simulink model "arlht_lu"  (R2020a)
settings: Solver=FixedStepDiscrete  StartTime=0.0  StopTime=inf  RelTol=1e-3
InitFcn:
  | % Clear workspace
  | clc; clear; close all;
  | 
  | fs = 250e6;
  | 
  | % Set parameters
  | height = 768;
  | width = 1024;
  | sobelThreshold = 30;
  | dTheta = 180/104;
  | theta = (0:dTheta:180-dTheta);
  | 
  | % Derive variables
  | maxRho = ceil(sqrt((height/2)^2+(width/2)^2));
  | nRho = maxRho*2;
  | nTheta = length(theta);
  | 
  | % Read in image and resize
  | I = imread('chess.jpg');
  | Ir = imresize(I, [height, width]);
  | 
  | % Get greyscale
  | Y = rgb2gray(Ir);
  | 
  | % Get Sobel and Gradient
  | [edge, dir, mag] = SobelEdge(Y, 100);
  | dirNew = floor(dir/dTheta)*dTheta;
  | simDirNew = dirNew*2^16;
  | simDirNew(edge==0) = 255*2^16;
  | 
  | % Create input array
  | inarray = uint32(simDirNew);
StopFcn:
  | [hps, Aopt, rbm] = ARLHT(edge, dirNew, dTheta, 1, 0, 4);
  | plot3DHPS(hps);
  | 
  | simHps = reshape(out.simout, [nRho, nTheta]);
  | plot3DHPS(simHps);
values from neighbouring files (symbols this model uses):
  dir = rad2deg(atan(Gy./Gx))    [SobelEdge.m]
libraries: simulink x53, hdlsllib x37, library x3, dspsrcs4 x1
(part 2 of 2)

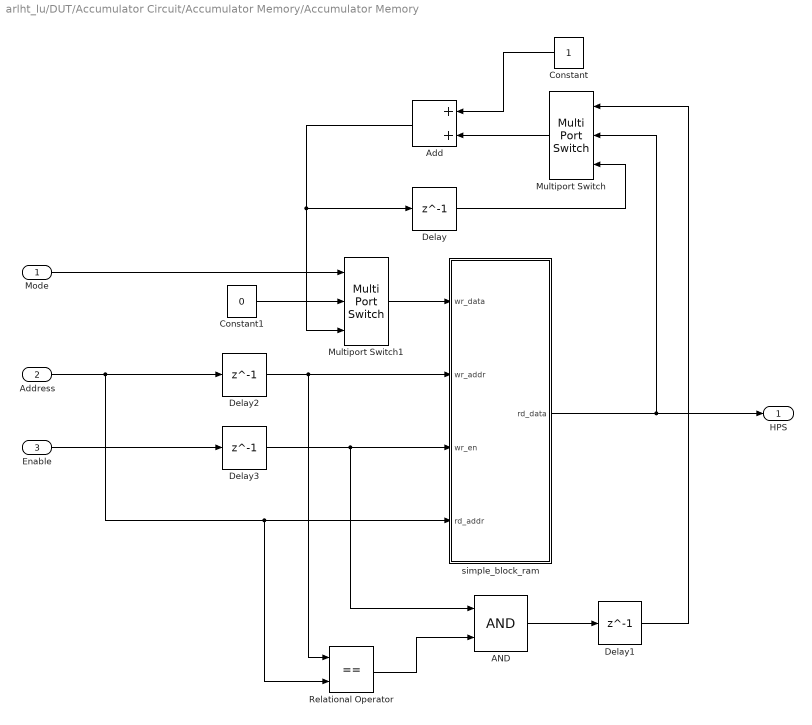
== system arlht_lu/DUT/Accumulator Circuit/Accumulator Memory/Accumulator Memory ==
  Mode : Inport
  Address : Inport  Port=2
  Enable : Inport  Port=3
  AND : Logic  IconShape=distinctive  AllPortsSameDT=off  OutDataTypeStr=boolean
  Add : Sum  OutDataTypeStr=fixdt(0,rhoBits,0)
  Constant : Constant  OutDataTypeStr=fixdt(0,1,0)  SampleTime=-1
  Constant1 : Constant  Value=0  OutDataTypeStr=fixdt(0,rhoBits,0)  SampleTime=-1
  Delay{,1..3} (4 alike) : Delay  DelayLength=1
  Multiport Switch : MultiPortSwitch  DataPortOrder=Zero-based contiguous  Inputs=2  zeroidx=on
  Multiport Switch1 : MultiPortSwitch  DataPortOrder=Zero-based contiguous  Inputs=2  zeroidx=on
  Relational Operator : RelationalOperator  Operator===  OutDataTypeStr=boolean  RndMeth=Simplest
  simple_block_ram : Subsystem  VariantControl=other_bits  mask{b=rhoBits, d=nRho*nTheta/kTheta, b_hidden=36, d_hidden=33280}
      mask prompts: b "Data width:"; d "Depth:"
      mask init: same as arlht_lu/DUT/RBM Circuit/Accumulator Memory/simple_block_ram
  HPS : Outport
  wires:
  Mode/1 -> Multiport Switch1/1
  Multiport Switch1/1 -> simple_block_ram/1(wr_data)
  Address/1 -> Relational Operator/2, simple_block_ram/4(rd_addr), Delay2/1
  simple_block_ram/1(rd_data) -> HPS/1, Multiport Switch/2
  AND/1 -> Delay1/1
  Delay/1 -> Multiport Switch/3
  Multiport Switch/1 -> Add/2
  Delay2/1 -> Relational Operator/1, simple_block_ram/2(wr_addr)
  Constant/1 -> Add/1
  Constant1/1 -> Multiport Switch1/2
  Add/1 -> Multiport Switch1/3, Delay/1
  Delay3/1 -> AND/1, simple_block_ram/3(wr_en)
  Relational Operator/1 -> AND/2
  Enable/1 -> Delay3/1
  Delay1/1 -> Multiport Switch/1

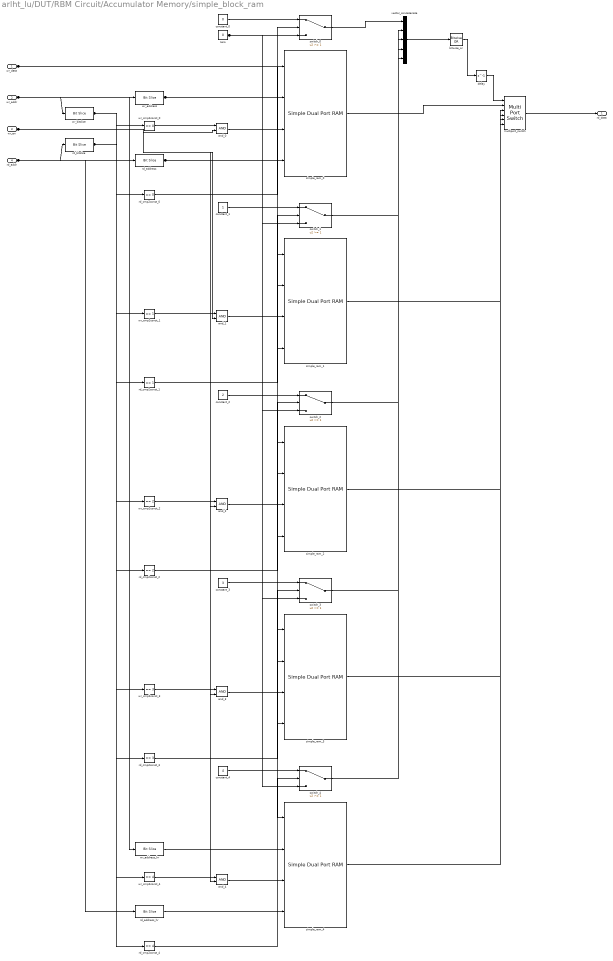
== system arlht_lu/DUT/RBM Circuit/Accumulator Memory/simple_block_ram ==
  wr_data : Inport
  wr_addr : Inport  Port=2
  wr_en : Inport  Port=3
  rd_addr : Inport  Port=4
  and_{0..4} (5 alike) : Logic  AllPortsSameDT=off  OutDataTypeStr=boolean
  bitwise_or : simulink/Logic and Bit Operations/Bitwise Operator  logicop=OR  UseBitMask=off  BitMask=bin2dec('11011001')  BitMaskRealWorld=Stored Integer
  constant_0 : Constant  Value=0  OutDataTypeStr=fixdt(0, 5, 0)  SampleTime=-1
  constant_1 : Constant  OutDataTypeStr=fixdt(0, 5, 0)  SampleTime=-1
  constant_2 : Constant  Value=2  OutDataTypeStr=fixdt(0, 5, 0)  SampleTime=-1
  constant_3 : Constant  Value=3  OutDataTypeStr=fixdt(0, 5, 0)  SampleTime=-1
  constant_4 : Constant  Value=4  OutDataTypeStr=fixdt(0, 5, 0)  SampleTime=-1
  delay : Delay  DelayLength=1
  multiport_switch : MultiPortSwitch  DataPortOrder=Zero-based contiguous  Inputs=5  zeroidx=on
  rd_address : hdlsllib/Logic and Bit Operations/Bit Slice  lidx=14  ridx=0
      settings: SourceProductBaseCode=SL
  rd_address_hr : hdlsllib/Logic and Bit Operations/Bit Slice  lidx=13  ridx=0
      settings: SourceProductBaseCode=SL
  rd_bitslice : hdlsllib/Logic and Bit Operations/Bit Slice  lidx=17  ridx=15
      settings: SourceProductBaseCode=SL
  rd_cmp2const_0 : simulink/Logic and Bit Operations/Compare To Constant  relop===  const=0  OutDataTypeStr=boolean
  rd_cmp2const_1 : simulink/Logic and Bit Operations/Compare To Constant  relop===  const=1  OutDataTypeStr=boolean
  rd_cmp2const_2 : simulink/Logic and Bit Operations/Compare To Constant  relop===  const=2  OutDataTypeStr=boolean
  rd_cmp2const_3 : simulink/Logic and Bit Operations/Compare To Constant  relop===  const=3  OutDataTypeStr=boolean
  rd_cmp2const_4 : simulink/Logic and Bit Operations/Compare To Constant  relop===  const=4  OutDataTypeStr=boolean
  simple_ram_{0..3} (4 alike) : hdlsllib/HDL RAMs/Simple Dual Port RAM  ram_size=15
      settings: SourceProductBaseCode=SL
  simple_ram_4 : hdlsllib/HDL RAMs/Simple Dual Port RAM  ram_size=14
      settings: SourceProductBaseCode=SL
  switch_{0..4} (5 alike) : Switch  Threshold=1
  vector_concatenate : Concatenate  NumInputs=5
  wr_address : hdlsllib/Logic and Bit Operations/Bit Slice  lidx=14  ridx=0
      settings: SourceProductBaseCode=SL
  wr_address_hr : hdlsllib/Logic and Bit Operations/Bit Slice  lidx=13  ridx=0
      settings: SourceProductBaseCode=SL
  wr_bitslice : hdlsllib/Logic and Bit Operations/Bit Slice  lidx=17  ridx=15
      settings: SourceProductBaseCode=SL
  wr_cmp2const_0 : simulink/Logic and Bit Operations/Compare To Constant  relop===  const=0  OutDataTypeStr=boolean
  wr_cmp2const_1 : simulink/Logic and Bit Operations/Compare To Constant  relop===  const=1  OutDataTypeStr=boolean
  wr_cmp2const_2 : simulink/Logic and Bit Operations/Compare To Constant  relop===  const=2  OutDataTypeStr=boolean
  wr_cmp2const_3 : simulink/Logic and Bit Operations/Compare To Constant  relop===  const=3  OutDataTypeStr=boolean
  wr_cmp2const_4 : simulink/Logic and Bit Operations/Compare To Constant  relop===  const=4  OutDataTypeStr=boolean
  zero : Constant  Value=0  OutDataTypeStr=fixdt(0, 5, 0)  SampleTime=-1
  rd_data : Outport
  wires:
  wr_data/1 -> simple_ram_0/1, simple_ram_1/1, simple_ram_2/1, simple_ram_3/1, simple_ram_4/1
  wr_address/1 -> simple_ram_0/2, simple_ram_1/2, simple_ram_2/2, simple_ram_3/2
  rd_address/1 -> simple_ram_0/4, simple_ram_1/4, simple_ram_2/4, simple_ram_3/4
  constant_0/1 -> switch_0/1
  zero/1 -> switch_0/3, switch_1/3, switch_2/3, switch_3/3, switch_4/3
  switch_0/1 -> vector_concatenate/1
  simple_ram_0/1 -> multiport_switch/2
  wr_bitslice/1 -> wr_cmp2const_0/1, wr_cmp2const_1/1, wr_cmp2const_2/1, wr_cmp2const_3/1, wr_cmp2const_4/1
  rd_bitslice/1 -> rd_cmp2const_0/1, rd_cmp2const_1/1, rd_cmp2const_2/1, rd_cmp2const_3/1, rd_cmp2const_4/1
  wr_en/1 -> and_0/2, and_1/2, and_2/2, and_3/2, and_4/2
  and_0/1 -> simple_ram_0/3
  wr_cmp2const_0/1 -> and_0/1
  rd_cmp2const_0/1 -> switch_0/2
  constant_1/1 -> switch_1/1
  switch_1/1 -> vector_concatenate/2
  simple_ram_1/1 -> multiport_switch/3
  and_1/1 -> simple_ram_1/3
  wr_cmp2const_1/1 -> and_1/1
  rd_cmp2const_1/1 -> switch_1/2
  constant_2/1 -> switch_2/1
  switch_2/1 -> vector_concatenate/3
  simple_ram_2/1 -> multiport_switch/4
  and_2/1 -> simple_ram_2/3
  wr_cmp2const_2/1 -> and_2/1
  rd_cmp2const_2/1 -> switch_2/2
  constant_3/1 -> switch_3/1
  switch_3/1 -> vector_concatenate/4
  simple_ram_3/1 -> multiport_switch/5
  and_3/1 -> simple_ram_3/3
  wr_cmp2const_3/1 -> and_3/1
  rd_cmp2const_3/1 -> switch_3/2
  constant_4/1 -> switch_4/1
  switch_4/1 -> vector_concatenate/5
  simple_ram_4/1 -> multiport_switch/6
  and_4/1 -> simple_ram_4/3
  wr_cmp2const_4/1 -> and_4/1
  rd_cmp2const_4/1 -> switch_4/2
  rd_addr/1 -> rd_bitslice/1, rd_address/1, rd_address_hr/1
  wr_addr/1 -> wr_bitslice/1, wr_address/1, wr_address_hr/1
  vector_concatenate/1 -> bitwise_or/1
  bitwise_or/1 -> delay/1
  delay/1 -> multiport_switch/1
  multiport_switch/1 -> rd_data/1
  wr_address_hr/1 -> simple_ram_4/2
  rd_address_hr/1 -> simple_ram_4/4

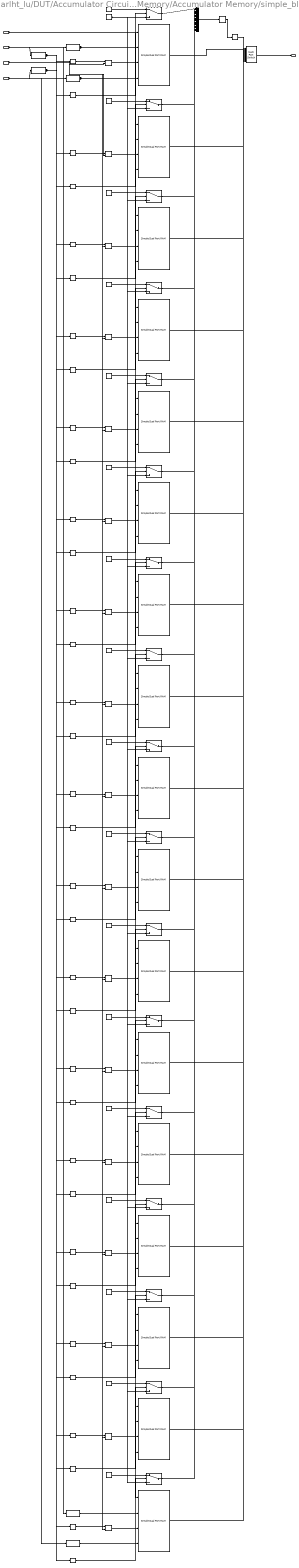
== system arlht_lu/DUT/Accumulator Circuit/Accumulator Memory/Accumulator Memory/simple_block_ram ==
  wr_data : Inport
  wr_addr : Inport  Port=2
  wr_en : Inport  Port=3
  rd_addr : Inport  Port=4
  and_{0..16} (17 alike) : Logic  AllPortsSameDT=off  OutDataTypeStr=boolean
  bitwise_or : simulink/Logic and Bit Operations/Bitwise Operator  logicop=OR  UseBitMask=off  BitMask=bin2dec('11011001')  BitMaskRealWorld=Stored Integer
  constant_0 : Constant  Value=0  OutDataTypeStr=fixdt(0, 17, 0)  SampleTime=-1
  constant_1 : Constant  OutDataTypeStr=fixdt(0, 17, 0)  SampleTime=-1
  constant_10 : Constant  Value=10  OutDataTypeStr=fixdt(0, 17, 0)  SampleTime=-1
  constant_11 : Constant  Value=11  OutDataTypeStr=fixdt(0, 17, 0)  SampleTime=-1
  constant_12 : Constant  Value=12  OutDataTypeStr=fixdt(0, 17, 0)  SampleTime=-1
  constant_13 : Constant  Value=13  OutDataTypeStr=fixdt(0, 17, 0)  SampleTime=-1
  constant_14 : Constant  Value=14  OutDataTypeStr=fixdt(0, 17, 0)  SampleTime=-1
  constant_15 : Constant  Value=15  OutDataTypeStr=fixdt(0, 17, 0)  SampleTime=-1
  constant_16 : Constant  Value=16  OutDataTypeStr=fixdt(0, 17, 0)  SampleTime=-1
  constant_2 : Constant  Value=2  OutDataTypeStr=fixdt(0, 17, 0)  SampleTime=-1
  constant_3 : Constant  Value=3  OutDataTypeStr=fixdt(0, 17, 0)  SampleTime=-1
  constant_4 : Constant  Value=4  OutDataTypeStr=fixdt(0, 17, 0)  SampleTime=-1
  constant_5 : Constant  Value=5  OutDataTypeStr=fixdt(0, 17, 0)  SampleTime=-1
  constant_6 : Constant  Value=6  OutDataTypeStr=fixdt(0, 17, 0)  SampleTime=-1
  constant_7 : Constant  Value=7  OutDataTypeStr=fixdt(0, 17, 0)  SampleTime=-1
  constant_8 : Constant  Value=8  OutDataTypeStr=fixdt(0, 17, 0)  SampleTime=-1
  constant_9 : Constant  Value=9  OutDataTypeStr=fixdt(0, 17, 0)  SampleTime=-1
  delay : Delay  DelayLength=1
  multiport_switch : MultiPortSwitch  DataPortOrder=Zero-based contiguous  Inputs=17  zeroidx=on
  rd_address : hdlsllib/Logic and Bit Operations/Bit Slice  lidx=10  ridx=0
      settings: SourceProductBaseCode=SL
  rd_address_hr : hdlsllib/Logic and Bit Operations/Bit Slice  lidx=9  ridx=0
      settings: SourceProductBaseCode=SL
  rd_bitslice : hdlsllib/Logic and Bit Operations/Bit Slice  lidx=15  ridx=11
      settings: SourceProductBaseCode=SL
  rd_cmp2const_0 : simulink/Logic and Bit Operations/Compare To Constant  relop===  const=0  OutDataTypeStr=boolean
  rd_cmp2const_1 : simulink/Logic and Bit Operations/Compare To Constant  relop===  const=1  OutDataTypeStr=boolean
  rd_cmp2const_10 : simulink/Logic and Bit Operations/Compare To Constant  relop===  const=10  OutDataTypeStr=boolean
  rd_cmp2const_11 : simulink/Logic and Bit Operations/Compare To Constant  relop===  const=11  OutDataTypeStr=boolean
  rd_cmp2const_12 : simulink/Logic and Bit Operations/Compare To Constant  relop===  const=12  OutDataTypeStr=boolean
  rd_cmp2const_13 : simulink/Logic and Bit Operations/Compare To Constant  relop===  const=13  OutDataTypeStr=boolean
  rd_cmp2const_14 : simulink/Logic and Bit Operations/Compare To Constant  relop===  const=14  OutDataTypeStr=boolean
  rd_cmp2const_15 : simulink/Logic and Bit Operations/Compare To Constant  relop===  const=15  OutDataTypeStr=boolean
  rd_cmp2const_16 : simulink/Logic and Bit Operations/Compare To Constant  relop===  const=16  OutDataTypeStr=boolean
  rd_cmp2const_2 : simulink/Logic and Bit Operations/Compare To Constant  relop===  const=2  OutDataTypeStr=boolean
  rd_cmp2const_3 : simulink/Logic and Bit Operations/Compare To Constant  relop===  const=3  OutDataTypeStr=boolean
  rd_cmp2const_4 : simulink/Logic and Bit Operations/Compare To Constant  relop===  const=4  OutDataTypeStr=boolean
  rd_cmp2const_5 : simulink/Logic and Bit Operations/Compare To Constant  relop===  const=5  OutDataTypeStr=boolean
  rd_cmp2const_6 : simulink/Logic and Bit Operations/Compare To Constant  relop===  const=6  OutDataTypeStr=boolean
  rd_cmp2const_7 : simulink/Logic and Bit Operations/Compare To Constant  relop===  const=7  OutDataTypeStr=boolean
  rd_cmp2const_8 : simulink/Logic and Bit Operations/Compare To Constant  relop===  const=8  OutDataTypeStr=boolean
  rd_cmp2const_9 : simulink/Logic and Bit Operations/Compare To Constant  relop===  const=9  OutDataTypeStr=boolean
  simple_ram_{0..15} (16 alike) : hdlsllib/HDL RAMs/Simple Dual Port RAM  ram_size=11
      settings: SourceProductBaseCode=SL
  simple_ram_16 : hdlsllib/HDL RAMs/Simple Dual Port RAM  ram_size=10
      settings: SourceProductBaseCode=SL
  switch_{0..16} (17 alike) : Switch  Threshold=1
  vector_concatenate : Concatenate  NumInputs=17
  wr_address : hdlsllib/Logic and Bit Operations/Bit Slice  lidx=10  ridx=0
      settings: SourceProductBaseCode=SL
  wr_address_hr : hdlsllib/Logic and Bit Operations/Bit Slice  lidx=9  ridx=0
      settings: SourceProductBaseCode=SL
  wr_bitslice : hdlsllib/Logic and Bit Operations/Bit Slice  lidx=15  ridx=11
      settings: SourceProductBaseCode=SL
  wr_cmp2const_0 : simulink/Logic and Bit Operations/Compare To Constant  relop===  const=0  OutDataTypeStr=boolean
  wr_cmp2const_1 : simulink/Logic and Bit Operations/Compare To Constant  relop===  const=1  OutDataTypeStr=boolean
  wr_cmp2const_10 : simulink/Logic and Bit Operations/Compare To Constant  relop===  const=10  OutDataTypeStr=boolean
  wr_cmp2const_11 : simulink/Logic and Bit Operations/Compare To Constant  relop===  const=11  OutDataTypeStr=boolean
  wr_cmp2const_12 : simulink/Logic and Bit Operations/Compare To Constant  relop===  const=12  OutDataTypeStr=boolean
  wr_cmp2const_13 : simulink/Logic and Bit Operations/Compare To Constant  relop===  const=13  OutDataTypeStr=boolean
  wr_cmp2const_14 : simulink/Logic and Bit Operations/Compare To Constant  relop===  const=14  OutDataTypeStr=boolean
  wr_cmp2const_15 : simulink/Logic and Bit Operations/Compare To Constant  relop===  const=15  OutDataTypeStr=boolean
  wr_cmp2const_16 : simulink/Logic and Bit Operations/Compare To Constant  relop===  const=16  OutDataTypeStr=boolean
  wr_cmp2const_2 : simulink/Logic and Bit Operations/Compare To Constant  relop===  const=2  OutDataTypeStr=boolean
  wr_cmp2const_3 : simulink/Logic and Bit Operations/Compare To Constant  relop===  const=3  OutDataTypeStr=boolean
  wr_cmp2const_4 : simulink/Logic and Bit Operations/Compare To Constant  relop===  const=4  OutDataTypeStr=boolean
  wr_cmp2const_5 : simulink/Logic and Bit Operations/Compare To Constant  relop===  const=5  OutDataTypeStr=boolean
  wr_cmp2const_6 : simulink/Logic and Bit Operations/Compare To Constant  relop===  const=6  OutDataTypeStr=boolean
  wr_cmp2const_7 : simulink/Logic and Bit Operations/Compare To Constant  relop===  const=7  OutDataTypeStr=boolean
  wr_cmp2const_8 : simulink/Logic and Bit Operations/Compare To Constant  relop===  const=8  OutDataTypeStr=boolean
  wr_cmp2const_9 : simulink/Logic and Bit Operations/Compare To Constant  relop===  const=9  OutDataTypeStr=boolean
  zero : Constant  Value=0  OutDataTypeStr=fixdt(0, 17, 0)  SampleTime=-1
  rd_data : Outport
  wires:
  wr_data/1 -> simple_ram_0/1, simple_ram_1/1, simple_ram_2/1, simple_ram_3/1, simple_ram_4/1, simple_ram_5/1, simple_ram_6/1, simple_ram_7/1, simple_ram_8/1, simple_ram_9/1, simple_ram_10/1, simple_ram_11/1, simple_ram_12/1, simple_ram_13/1, simple_ram_14/1, simple_ram_15/1, simple_ram_16/1
  wr_address/1 -> simple_ram_0/2, simple_ram_1/2, simple_ram_2/2, simple_ram_3/2, simple_ram_4/2, simple_ram_5/2, simple_ram_6/2, simple_ram_7/2, simple_ram_8/2, simple_ram_9/2, simple_ram_10/2, simple_ram_11/2, simple_ram_12/2, simple_ram_13/2, simple_ram_14/2, simple_ram_15/2
  rd_address/1 -> simple_ram_0/4, simple_ram_1/4, simple_ram_2/4, simple_ram_3/4, simple_ram_4/4, simple_ram_5/4, simple_ram_6/4, simple_ram_7/4, simple_ram_8/4, simple_ram_9/4, simple_ram_10/4, simple_ram_11/4, simple_ram_12/4, simple_ram_13/4, simple_ram_14/4, simple_ram_15/4
  constant_0/1 -> switch_0/1
  zero/1 -> switch_0/3, switch_1/3, switch_2/3, switch_3/3, switch_4/3, switch_5/3, switch_6/3, switch_7/3, switch_8/3, switch_9/3, switch_10/3, switch_11/3, switch_12/3, switch_13/3, switch_14/3, switch_15/3, switch_16/3
  switch_0/1 -> vector_concatenate/1
  simple_ram_0/1 -> multiport_switch/2
  wr_bitslice/1 -> wr_cmp2const_0/1, wr_cmp2const_1/1, wr_cmp2const_2/1, wr_cmp2const_3/1, wr_cmp2const_4/1, wr_cmp2const_5/1, wr_cmp2const_6/1, wr_cmp2const_7/1, wr_cmp2const_8/1, wr_cmp2const_9/1, wr_cmp2const_10/1, wr_cmp2const_11/1, wr_cmp2const_12/1, wr_cmp2const_13/1, wr_cmp2const_14/1, wr_cmp2const_15/1, wr_cmp2const_16/1
  rd_bitslice/1 -> rd_cmp2const_0/1, rd_cmp2const_1/1, rd_cmp2const_2/1, rd_cmp2const_3/1, rd_cmp2const_4/1, rd_cmp2const_5/1, rd_cmp2const_6/1, rd_cmp2const_7/1, rd_cmp2const_8/1, rd_cmp2const_9/1, rd_cmp2const_10/1, rd_cmp2const_11/1, rd_cmp2const_12/1, rd_cmp2const_13/1, rd_cmp2const_14/1, rd_cmp2const_15/1, rd_cmp2const_16/1
  wr_en/1 -> and_0/2, and_1/2, and_2/2, and_3/2, and_4/2, and_5/2, and_6/2, and_7/2, and_8/2, and_9/2, and_10/2, and_11/2, and_12/2, and_13/2, and_14/2, and_15/2, and_16/2
  and_0/1 -> simple_ram_0/3
  wr_cmp2const_0/1 -> and_0/1
  rd_cmp2const_0/1 -> switch_0/2
  constant_1/1 -> switch_1/1
  switch_1/1 -> vector_concatenate/2
  simple_ram_1/1 -> multiport_switch/3
  and_1/1 -> simple_ram_1/3
  wr_cmp2const_1/1 -> and_1/1
  rd_cmp2const_1/1 -> switch_1/2
  constant_2/1 -> switch_2/1
  switch_2/1 -> vector_concatenate/3
  simple_ram_2/1 -> multiport_switch/4
  and_2/1 -> simple_ram_2/3
  wr_cmp2const_2/1 -> and_2/1
  rd_cmp2const_2/1 -> switch_2/2
  constant_3/1 -> switch_3/1
  switch_3/1 -> vector_concatenate/4
  simple_ram_3/1 -> multiport_switch/5
  and_3/1 -> simple_ram_3/3
  wr_cmp2const_3/1 -> and_3/1
  rd_cmp2const_3/1 -> switch_3/2
  constant_4/1 -> switch_4/1
  switch_4/1 -> vector_concatenate/5
  simple_ram_4/1 -> multiport_switch/6
  and_4/1 -> simple_ram_4/3
  wr_cmp2const_4/1 -> and_4/1
  rd_cmp2const_4/1 -> switch_4/2
  constant_5/1 -> switch_5/1
  switch_5/1 -> vector_concatenate/6
  simple_ram_5/1 -> multiport_switch/7
  and_5/1 -> simple_ram_5/3
  wr_cmp2const_5/1 -> and_5/1
  rd_cmp2const_5/1 -> switch_5/2
  constant_6/1 -> switch_6/1
  switch_6/1 -> vector_concatenate/7
  simple_ram_6/1 -> multiport_switch/8
  and_6/1 -> simple_ram_6/3
  wr_cmp2const_6/1 -> and_6/1
  rd_cmp2const_6/1 -> switch_6/2
  constant_7/1 -> switch_7/1
  switch_7/1 -> vector_concatenate/8
  simple_ram_7/1 -> multiport_switch/9
  and_7/1 -> simple_ram_7/3
  wr_cmp2const_7/1 -> and_7/1
  rd_cmp2const_7/1 -> switch_7/2
  constant_8/1 -> switch_8/1
  switch_8/1 -> vector_concatenate/9
  simple_ram_8/1 -> multiport_switch/10
  and_8/1 -> simple_ram_8/3
  wr_cmp2const_8/1 -> and_8/1
  rd_cmp2const_8/1 -> switch_8/2
  constant_9/1 -> switch_9/1
  switch_9/1 -> vector_concatenate/10
  simple_ram_9/1 -> multiport_switch/11
  and_9/1 -> simple_ram_9/3
  wr_cmp2const_9/1 -> and_9/1
  rd_cmp2const_9/1 -> switch_9/2
  constant_10/1 -> switch_10/1
  switch_10/1 -> vector_concatenate/11
  simple_ram_10/1 -> multiport_switch/12
  and_10/1 -> simple_ram_10/3
  wr_cmp2const_10/1 -> and_10/1
  rd_cmp2const_10/1 -> switch_10/2
  constant_11/1 -> switch_11/1
  switch_11/1 -> vector_concatenate/12
  simple_ram_11/1 -> multiport_switch/13
  and_11/1 -> simple_ram_11/3
  wr_cmp2const_11/1 -> and_11/1
  rd_cmp2const_11/1 -> switch_11/2
  constant_12/1 -> switch_12/1
  switch_12/1 -> vector_concatenate/13
  simple_ram_12/1 -> multiport_switch/14
  and_12/1 -> simple_ram_12/3
  wr_cmp2const_12/1 -> and_12/1
  rd_cmp2const_12/1 -> switch_12/2
  constant_13/1 -> switch_13/1
  switch_13/1 -> vector_concatenate/14
  simple_ram_13/1 -> multiport_switch/15
  and_13/1 -> simple_ram_13/3
  wr_cmp2const_13/1 -> and_13/1
  rd_cmp2const_13/1 -> switch_13/2
  constant_14/1 -> switch_14/1
  switch_14/1 -> vector_concatenate/15
  simple_ram_14/1 -> multiport_switch/16
  and_14/1 -> simple_ram_14/3
  wr_cmp2const_14/1 -> and_14/1
  rd_cmp2const_14/1 -> switch_14/2
  constant_15/1 -> switch_15/1
  switch_15/1 -> vector_concatenate/16
  simple_ram_15/1 -> multiport_switch/17
  and_15/1 -> simple_ram_15/3
  wr_cmp2const_15/1 -> and_15/1
  rd_cmp2const_15/1 -> switch_15/2
  constant_16/1 -> switch_16/1
  switch_16/1 -> vector_concatenate/17
  simple_ram_16/1 -> multiport_switch/18
  and_16/1 -> simple_ram_16/3
  wr_cmp2const_16/1 -> and_16/1
  rd_cmp2const_16/1 -> switch_16/2
  rd_addr/1 -> rd_bitslice/1, rd_address/1, rd_address_hr/1
  wr_addr/1 -> wr_bitslice/1, wr_address/1, wr_address_hr/1
  vector_concatenate/1 -> bitwise_or/1
  bitwise_or/1 -> delay/1
  delay/1 -> multiport_switch/1
  multiport_switch/1 -> rd_data/1
  wr_address_hr/1 -> simple_ram_16/2
  rd_address_hr/1 -> simple_ram_16/4

== matlab function arlht_lu/DUT/Accumulator Circuit/MATLAB Function ==
  data: sof input; mode output; rho_address output; theta_address output; eof input; ntheta input; nrho input; ktheta input; clear output; valid output; debug_state output
function [mode, rho_address, theta_address, clear, valid, debug_state] = fcn(sof, eof, ntheta, nrho, ktheta)

IDLE = fi(0, 0, 2, 0);
VOTE = fi(1, 0, 2, 0);
READ = fi(2, 0, 2, 0);
CLEAR = fi(3, 0, 2, 0);

persistent current_state;
persistent rho_count;
persistent theta_count;
persistent k_count;

if isempty(current_state)
    current_state = IDLE;
end

if isempty(rho_count)
    rho_count = fi(0, 0, 16, 0);
end

if isempty(theta_count)
    theta_count = fi(0, 0, 8, 0);
end

if isempty(k_count)
    k_count = fi(0, 0, 8, 0);
end

switch current_state
    case IDLE
        mode = false;
        valid = false;
        clear = false;
        rho_address = rho_count;
        theta_address = theta_count;
        debug_state = IDLE;
        
        if sof
            current_state = VOTE;
        else
            current_state = IDLE;
        end
        
    case VOTE
        mode = true;
        valid = false;
        clear = false;
        rho_address = rho_count;
        theta_address = theta_count;
        debug_state = VOTE;
        
        if eof
            current_state = READ;
        else
            current_state = VOTE;
        end
        
    case READ
        mode = false;
        valid = true;
        clear = false;
        rho_address = rho_count;
        theta_address = theta_count;
        debug_state = READ;
        
        if (rho_count >= nrho-1)
            rho_count = fi(0, 0, 16, 0);
            if (theta_count >= ntheta-1)
                theta_count = fi(0, 0, 8, 0);
                if (k_count >= ktheta-2)
                    k_count = fi(0, 0, 8, 0);
                    current_state = CLEAR;
                else
                    k_count = fi(k_count + 1, 0, 8, 0);
                    current_state = READ;
                end
            else
                theta_count = fi(theta_count + 1, 0, 8, 0);
                current_state = READ;
            end
        else
            rho_count = fi(rho_count + 1, 0, 16, 0);
            current_state = READ;
        end
        
    case CLEAR
        mode = false;
        valid = true;
        clear = true;
        rho_address = rho_count;
        theta_address = theta_count;
        debug_state = CLEAR;
        
        if (rho_count >= nrho-1)
            rho_count = fi(0, 0, 16, 0);
            if (theta_count >= ntheta-1)
                theta_count = fi(0, 0, 8, 0);
                current_state = IDLE;
            else
                theta_count = fi(theta_count + 1, 0, 8, 0);
                current_state = CLEAR;
            end
        else
            rho_count = fi(rho_count + 1, 0, 16, 0);
            current_state = CLEAR;
        end
        
    otherwise
        mode = false;
        valid = false;
        clear = false;
        rho_address = rho_count;
        theta_address = theta_count;
        debug_state = IDLE;
        
        current_state = IDLE;
        
end

== matlab function arlht_lu/DUT/RBM Circuit/RBM Controller ==
  data: sof input; mode output; rho_address output; theta_address output; eof input; ntheta input; nrho input; clear output; debug_state output
function [mode, rho_address, theta_address, clear, debug_state] = fcn(sof, eof, ntheta, nrho)

IDLE = fi(0, 0, 2, 0);
VOTE = fi(1, 0, 2, 0);
CLEAR = fi(2, 0, 2, 0);

persistent current_state;
persistent rho_count;
persistent theta_count;

if isempty(current_state)
    current_state = IDLE;
end

if isempty(rho_count)
    rho_count = fi(0, 0, 16, 0);
end

if isempty(theta_count)
    theta_count = fi(0, 0, 8, 0);
end

switch current_state
    case IDLE
        mode = false;
        clear = false;
        rho_address = rho_count;
        theta_address = theta_count;
        debug_state = IDLE;
        
        if sof
            current_state = VOTE;
        else
            current_state = IDLE;
        end
        
    case VOTE
        mode = true;
        clear = false;
        rho_address = rho_count;
        theta_address = theta_count;
        debug_state = VOTE;
        
        if eof
            current_state = CLEAR;
        else
            current_state = VOTE;
        end
        
    case CLEAR
        mode = false;
        clear = true;
        rho_address = rho_count;
        theta_address = theta_count;
        debug_state = CLEAR;
        
        if (rho_count >= nrho-1)
            rho_count = fi(0, 0, 16, 0);
            if (theta_count >= ntheta-1)
                theta_count = fi(0, 0, 8, 0);
                current_state = IDLE;
            else
                theta_count = fi(theta_count + 1, 0, 8, 0);
                current_state = CLEAR;
            end
        else
            rho_count = fi(rho_count + 1, 0, 16, 0);
            current_state = CLEAR;
        end
        
    otherwise
        mode = false;
        clear = false;
        rho_address = rho_count;
        theta_address = theta_count;
        debug_state = IDLE
        
        current_state = IDLE;
        
end
